simulink model "mdl_tubing_simevents2"  (R2020b)
settings: Solver=VariableStepAuto  StartTime=0.0  StopTime=100.0  RelTol=1e-3
undefined symbols (not defined in the file): m, n
settings Model: Creator=natha  LastModifiedBy=natha

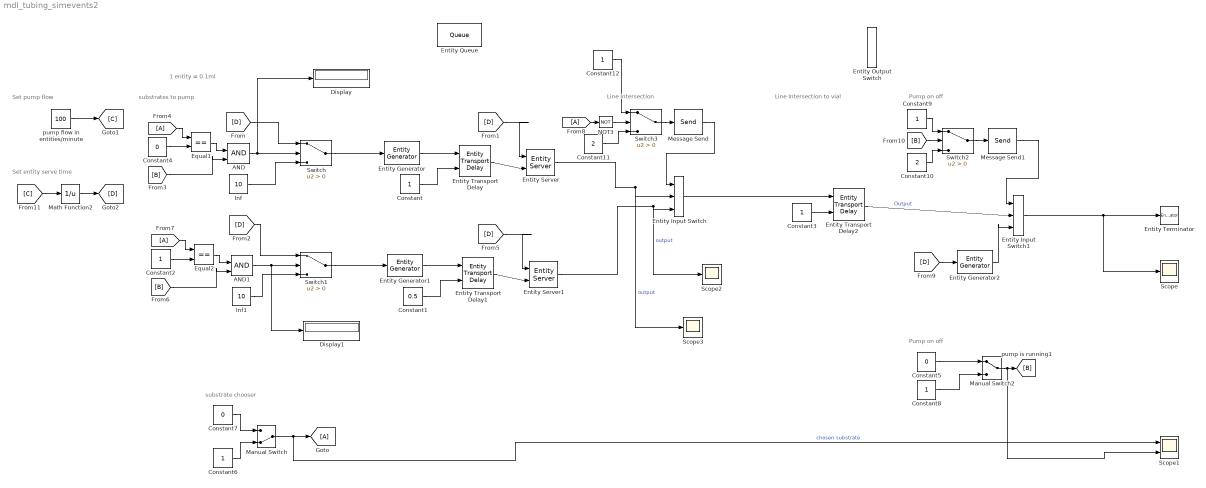
== system mdl_tubing_simevents2 ==
  note: Pump on off
  note: Line Intersection to vial
  note: Set pump flow
  note: 1 entity = 0.1ml
  note: substrate chooser
  note: substrates to pump
  note: Pump on off
  note: Line Intersection
  note: Set entity serve time
  AND : Logic  IconShape=distinctive  AllPortsSameDT=off  OutDataTypeStr=boolean
  AND1 : Logic  IconShape=distinctive  AllPortsSameDT=off  OutDataTypeStr=boolean
  Constant{,2..3,6,8..9,12} (7 alike) : Constant
  Constant1 : Constant  Value=0.5
  Constant10 : Constant  Value=2
  Constant11 : Constant  Value=2
  Constant4 : Constant  Value=0
  Constant5 : Constant  Value=0
  Constant7 : Constant  Value=0
  Display : Display
  Display1 : Display
  Entity Input Switch : EntityInputSwitch  InputPortMessageModes=m,m,m  OutputPortMessageModes=m  ActivePortSelection=Switch  SwitchingCriterion=From control port
      settings: InputPortMap=u0,u1,u2
  Entity Input Switch1 : EntityInputSwitch  InputPortMessageModes=m,m,m  OutputPortMessageModes=m  ActivePortSelection=Switch  SwitchingCriterion=From control port
      settings: InputPortMap=u0,u1,u2
  Entity Output Switch : EntityOutputSwitch  InputPortMessageModes=m  OutputPortMessageModes=m,m  SwitchAttributeName=Attribute1
  Entity Transport Delay : EntityTransportDelay  InputPortMessageModes=m,n  OutputPortMessageModes=m
  Entity Transport Delay1 : EntityTransportDelay  InputPortMessageModes=m,n  OutputPortMessageModes=m
  Entity Transport Delay2 : EntityTransportDelay  InputPortMessageModes=m,n  OutputPortMessageModes=m
  Entity Generator : EntityGenerator  OutputPortMessageModes=m  TimeSource=Signal port  GenerateEntityAtSimulationStart=off  AttributeName=Substrate  AttributeInitialValue=0  EntityType=Structured  EntityTypeName=Entity
      settings: InputPortMap=u1
  Entity Generator1 : EntityGenerator  OutputPortMessageModes=m  TimeSource=Signal port  GenerateEntityAtSimulationStart=off  AttributeName=Substrate  EntityType=Structured  EntityTypeName=Entity
      settings: InputPortMap=u1
  Entity Generator2 : EntityGenerator  OutputPortMessageModes=m  TimeSource=Signal port  GenerateEntityAtSimulationStart=off  AttributeName=Substrate  AttributeInitialValue=-1  EntityType=Structured  EntityTypeName=Entity
      settings: InputPortMap=u1
  Entity Queue : Queue  InputPortMessageModes=m  OutputPortMessageModes=m
  Entity Server : EntityServer  InputPortMessageModes=n,m  OutputPortMessageModes=m  Capacity=1  ServiceTimeSource=Signal port  ServiceTimeValue=0.3
      settings: InputPortMap=u0,u2
  Entity Server1 : EntityServer  InputPortMessageModes=n,m  OutputPortMessageModes=m  Capacity=1  ServiceTimeSource=Signal port  ServiceTimeValue=0.3
      settings: InputPortMap=u0,u2
  Entity Terminator : EntityTerminator  InputPortMessageModes=m
  Equal1 : RelationalOperator  Operator===  OutDataTypeStr=boolean  RndMeth=Simplest
  Equal2 : RelationalOperator  Operator===  OutDataTypeStr=boolean  RndMeth=Simplest
  Inf : Constant  Value=10  OutDataTypeStr=Inherit: Inherit via back propagation
  Inf1 : Constant  Value=10  OutDataTypeStr=Inherit: Inherit via back propagation
  Manual Switch : ManualSwitch  CurrentSetting=0
  Manual Switch2 : ManualSwitch
  Math Function2 : Math  Operator=reciprocal  SaturateOnIntegerOverflow=on
  Message Send : Send  OutputPortMessageModes=m
  Message Send1 : Send  OutputPortMessageModes=m
  NOT3 : Logic  Operator=NOT  IconShape=distinctive  AllPortsSameDT=off  OutDataTypeStr=boolean
  Scope : Scope
  Scope1 : Scope  NumInputPorts=2
  Scope2 : Scope
  Scope3 : Scope
  Switch{,1..3} (4 alike) : Switch  Criteria=u2 > Threshold
  pump flow in entities/minute : Constant  Value=100
  wires:
  Entity Transport Delay/1 -> Entity Server/2
  [D] -> Entity Server/1
  Constant4/1 -> Equal1/2
  Equal1/1 -> AND/1
  [B] -> AND/2
  [A] -> Equal1/1
  Manual Switch/1 -> Scope1/1, [A]  "chosen substrate"
  Constant6/1 -> Manual Switch/2
  Constant7/1 -> Manual Switch/1
  AND/1 -> Display/1, Switch/2
  Inf/1 -> Switch/3
  pump flow in entities/minute/1 -> [C]
  Constant/1 -> Entity Transport Delay/2
  Constant1/1 -> Entity Transport Delay1/2
  Inf1/1 -> Switch1/3
  AND1/1 -> Display1/1, Switch1/2
  [A] -> Equal2/1
  [B] -> AND1/2
  Equal2/1 -> AND1/1
  Constant2/1 -> Equal2/2
  [D] -> Entity Server1/1
  Entity Generator1/1 -> Entity Transport Delay1/1
  Entity Transport Delay1/1 -> Entity Server1/2
  Entity Transport Delay2/1 -> Entity Input Switch1/2  "Output"
  Entity Input Switch/1 -> Entity Transport Delay2/1
  Entity Server1/1 -> Scope2/1, Entity Input Switch/3  "output"
  Entity Server/1 -> Scope3/1, Entity Input Switch/2  "output"
  Constant3/1 -> Entity Transport Delay2/2
  Entity Generator2/1 -> Entity Input Switch1/3
  [D] -> Entity Generator2/1
  Manual Switch2/1 -> Scope1/2, [B]
  Constant5/1 -> Manual Switch2/1
  Constant8/1 -> Manual Switch2/2
  Entity Input Switch1/1 -> Scope/1, Entity Terminator/1
  [A] -> NOT3/1
  Message Send/1 -> Entity Input Switch/1
  [B] -> Switch2/2
  Message Send1/1 -> Entity Input Switch1/1
  Switch2/1 -> Message Send1/1
  Constant9/1 -> Switch2/1
  Constant10/1 -> Switch2/3
  Constant11/1 -> Switch3/3
  Constant12/1 -> Switch3/1
  Switch3/1 -> Message Send/1
  NOT3/1 -> Switch3/2
  [D] -> Switch/1
  [D] -> Switch1/1
  Math Function2/1 -> [D]
  [C] -> Math Function2/1
  Entity Generator/1 -> Entity Transport Delay/1
  Switch/1 -> Entity Generator/1
  Switch1/1 -> Entity Generator1/1
